simulink model "simu1_4"  (R2023a)
settings: Solver=VariableStepAuto  StartTime=0.0  StopTime=10.0  RelTol=1e-3
values from neighbouring files (symbols this model uses):
  C = 1    [mat1_4.m]
  L = 1    [mat1_4.m]
  R = 1    [mat1_4.m]
settings Model: Creator=lukas  LastModifiedBy=lukas

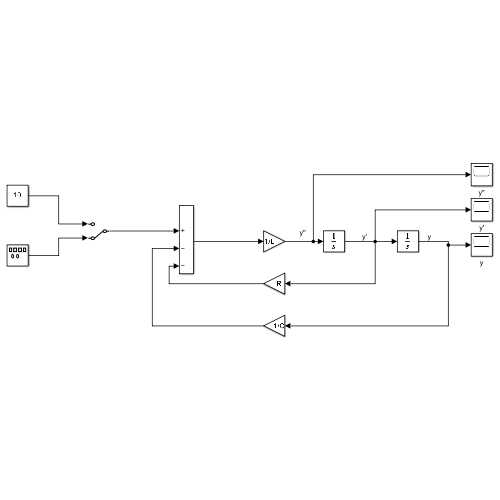
[thumbnail: Simulink's stored preview of the top-level diagram]
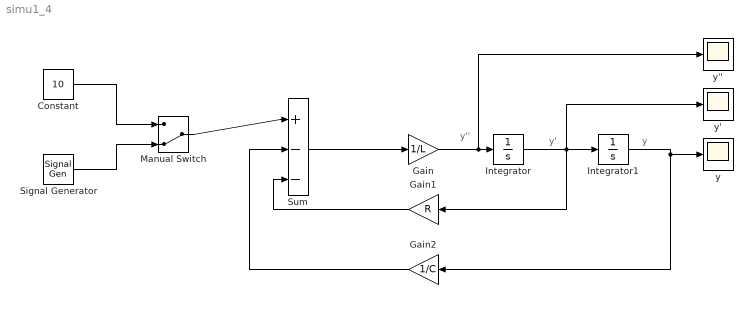
== system simu1_4 ==
  note: y
  note: y'
  note: y''
  Constant : Constant  Value=10
  Gain : Gain  Gain=1/L
  Gain1 : Gain  Gain=R
  Gain2 : Gain  Gain=1/C
  Integrator : Integrator
  Integrator1 : Integrator
  Manual Switch : ManualSwitch  CurrentSetting=0
  Signal Generator : SignalGenerator  Amplitude=10  Frequency=10  Units=rad/sec
  Sum : Sum  Inputs=|+--
  y : Scope
  y' : Scope
  y'' : Scope
  wires:
  Integrator/1 -> y'/1, Gain1/1, Integrator1/1
  Integrator1/1 -> y/1, Gain2/1
  Gain/1 -> y''/1, Integrator/1
  Sum/1 -> Gain/1
  Gain2/1 -> Sum/2
  Gain1/1 -> Sum/3
  Constant/1 -> Manual Switch/1
  Signal Generator/1 -> Manual Switch/2
  Manual Switch/1 -> Sum/1
